simulink model "control_foc"  (R2023b)
settings: Solver=FixedStepDiscrete  StartTime=0.0  StopTime=10.0  FixedStep=ControlFOC_Ts  RelTol=1e-3  EnableMultiTasking=on
model workspace (MAT data in the model file):
  ControlFOC_Ts = Simulink.Parameter
  ControlFOC_Ts.Value = 3.65714285714e-05
  ControlFOC_Ts.DataType = 'auto'
  ControlFOC_Ts.DocUnits = 's'
  ControlFOC_Ts.Complexity = 'real'
  ControlFOC_Ts.Dimensions = [1 1]
libraries: mcbcontrolslib x4, slpidlib x2, dspstat3 x2, simulink x1
settings Model: DataDictionary=EmbeddedBoardDD.sldd  Creator=ascalzo  LastModifiedBy=mfussi
settings SolverCC: AllowMultiTaskInputOutput=on  AutoInsertRateTranBlk=on  InsertRTBMode=Never (minimum delay)
settings DataIOCC: SaveOutput=off  SignalLogging=off  DSMLogging=off  SaveTime=off  ReturnWorkspaceOutputs=off
settings OptimizationCC: DefaultParameterBehavior=Inlined  DefaultUnderspecifiedDataType=single  StrengthReduction=on  PassReuseOutputArgsAs=Individual arguments  OptimizeBlockOrder=speed  OptimizationPriority=Speed  OptimizationCustomize=off  MultiThreadedLoops=on  EfficientTunableParamExpr=on
settings DebuggingCC: ParameterPrecisionLossMsg=none  UnconnectedInputMsg=warning  UnconnectedOutputMsg=warning  UnconnectedLineMsg=warning
settings HardwareCC: ProdBitPerPointer=32  ProdBitPerSizeT=32  ProdBitPerPtrDiffT=32  ProdLargestAtomicInteger=Long  ProdLargestAtomicFloat=Double  ProdWordSize=32  ProdHWDeviceType=ARM Compatible->ARM Cortex-M
settings ModelReferenceCC: UpdateModelReferenceTargets=Force  EnableRefExpFcnMdlSchedulingChecks=on
settings SFSimCC: MATLABDynamicMemAlloc=off
settings RTWCC: Description=Embedded Coder  SystemTargetFile=ert.tlc  GenCodeOnly=on  PackageGeneratedCodeAndArtifacts=on  PackageName=control_foc  TemplateMakefile=ert_default_tmf  TargetLang=C++  DLArmComputeVersion=19.05
settings CodeAppCC: ForceParamTrailComments=on  IgnoreCustomStorageClasses=off  MaxIdLength=60  OperatorAnnotations=on  SimulinkDataObjDesc=on  SFDataObjDesc=on  InsertBlockDesc=on
settings ERTTargetCC: TargetLangStandard=C++03 (ISO)  CodeReplacementLibrary=ARM Cortex-M,iCubTech  GenerateSampleERTMain=on  CodeInterfacePackaging=Reusable function  InlinedParameterPlacement=NonHierarchical  RootIOFormat=Structure reference  ERTCustomFileTemplate=example_file_process.tlc

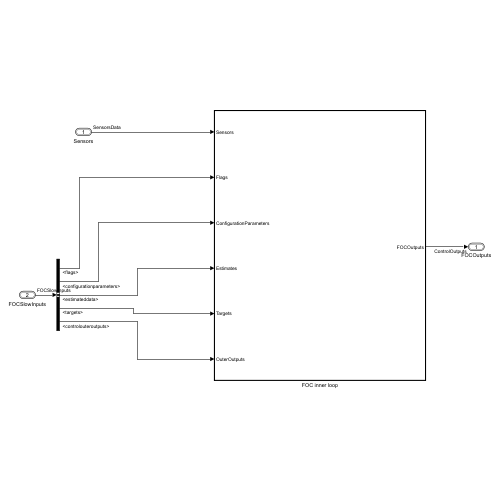
[thumbnail: Simulink's stored preview of the top-level diagram]
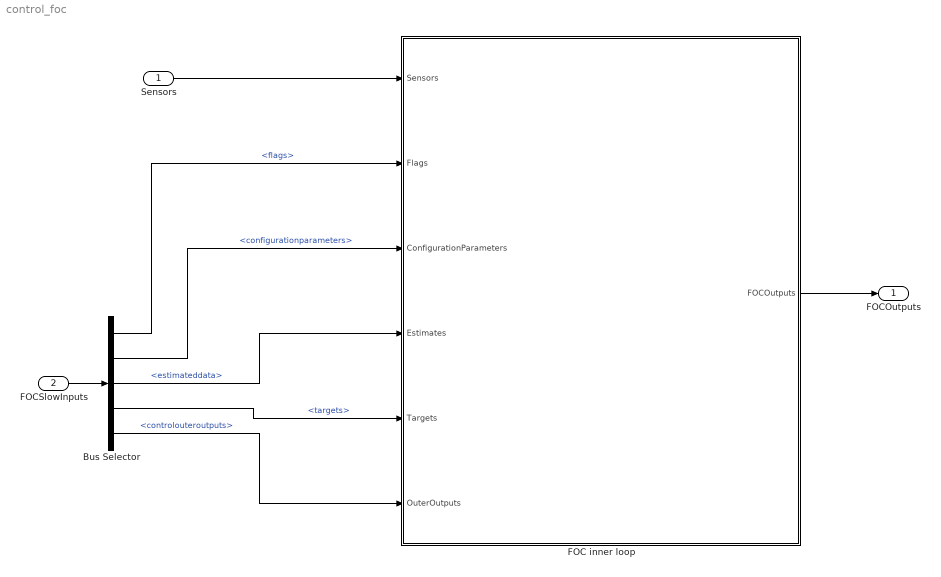
== system control_foc ==
  Sensors : Inport  OutDataTypeStr=Bus: SensorsData  BusOutputAsStruct=on
  FOCSlowInputs : Inport  Port=2  OutDataTypeStr=Bus: FOCSlowInputs  BusOutputAsStruct=on
  Bus Selector : BusSelector  OutputSignals=flags,configurationparameters,estimateddata,targets,controlouteroutputs
  FOC inner loop : Subsystem  TreatAsAtomicUnit=on  RTWFcnName=FOCInnerLoop
      settings: RTWFcnNameOpts=User specified  RTWFileNameOpts=Use function name  FunctionInterfaceSpec=Allow arguments (Optimized)
  FOCOutputs : Outport  OutDataTypeStr=Bus: ControlOutputs  BusOutputAsStruct=on
  wires:
  FOC inner loop/1(FOCOutputs) -> FOCOutputs/1
  FOCSlowInputs/1 -> Bus Selector/1
  Bus Selector/1 -> FOC inner loop/2(Flags)  "<flags>"
  Bus Selector/2 -> FOC inner loop/3(ConfigurationParameters)  "<configurationparameters>"
  Bus Selector/3 -> FOC inner loop/4(Estimates)  "<estimateddata>"
  Bus Selector/4 -> FOC inner loop/5(Targets)  "<targets>"
  Bus Selector/5 -> FOC inner loop/6(OuterOutputs)  "<controlouteroutputs>"
  Sensors/1 -> FOC inner loop/1(Sensors)

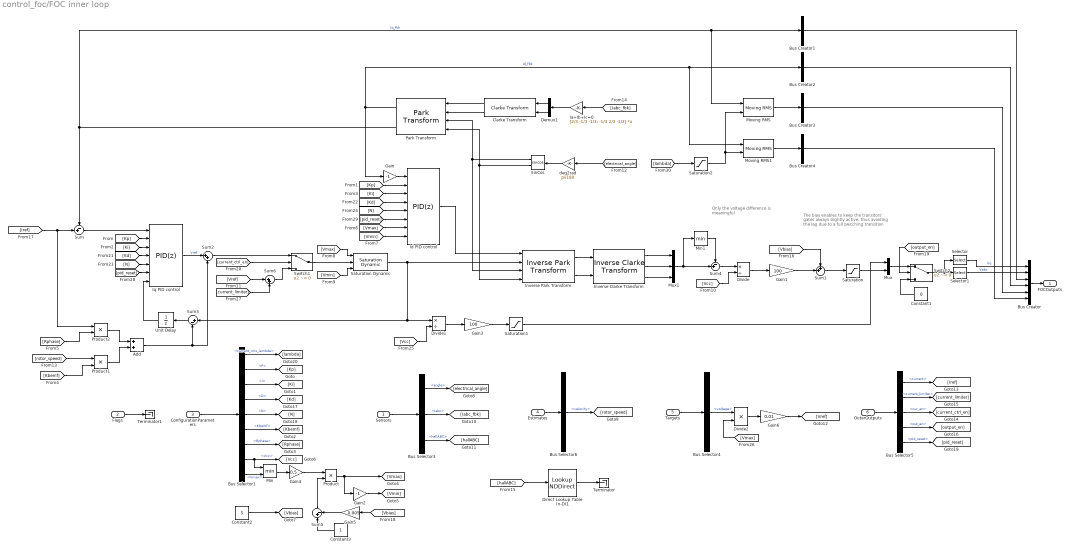
== system control_foc/FOC inner loop ==
  note: Only the voltage difference
      | is meaningful
  note: The bias enables to keep the transitors'
      | gates always slightly active, thus avoiding
      | the lag due to a full switching transition
  Sensors : Inport  OutDataTypeStr=Bus: SensorsData
  Flags : Inport  Port=2  OutDataTypeStr=Bus: Flags
  ConfigurationParameters : Inport  Port=3  OutDataTypeStr=Bus: ConfigurationParameters
  Estimates : Inport  Port=4  OutDataTypeStr=Bus: EstimatedData
  Targets : Inport  Port=5  OutDataTypeStr=Bus: Targets
  OuterOutputs : Inport  Port=6  OutDataTypeStr=Bus: ControlOuterOutputs
  Add : Sum
  Bus Creator : BusCreator  Inputs=6  OutDataTypeStr=Bus: ControlOutputs  NonVirtualBus=on
      settings: InheritFromInputs=off
  Bus Creator{1..4} (4 alike) : BusCreator  Inputs=1  OutDataTypeStr=Bus: MotorCurrent  NonVirtualBus=on
      settings: InheritFromInputs=off
  Bus Selector1 : BusSelector  OutputSignals=estimationconfig.current_rms_lambda,CurLoopPID.P,CurLoopPID.I,CurLoopPID.D,CurLoopPID.N,motorconfig.Kbemf,motorconfig.Rphase,motorconfig.Vcc,motorconfig.Vmax
  Bus Selector3 : BusSelector  OutputSignals=motorsensors.angle,motorsensors.Iabc,motorsensors.hallABC
  Bus Selector4 : BusSelector  OutputSignals=motorvoltage.voltage
  Bus Selector5 : BusSelector  OutputSignals=motorcurrent.current,current_limiter,cur_en,out_en,pid_reset
  Bus Selector6 : BusSelector  OutputSignals=jointvelocities.velocity
  Clarke Transform : mcbcontrolslib/Clarke Transform  VariantControl=Variant2  PhaseInput=Two inputs  EnPowerInv=off
  Constant1 : Constant  Value=0  OutDataTypeStr=single
  Constant2 : Constant  Value=5  OutDataTypeStr=single
  Constant3 : Constant  OutDataTypeStr=single
  Demux1 : Demux  Outputs=2
  Direct Lookup Table (n-D)1 : LookupNDDirect  NumberOfTableDimensions=1  Table=[-1,270,150,210,30,330,90,-1]  RemoveProtectionInput=on  TableDataTypeStr=single
  Divide : Product  Inputs=*/
  Divide1 : Product  Inputs=*/
  Divide2 : Product
  Gain : Gain  Gain=-1
  Gain1 : Gain  Gain=100
  Gain2 : Gain  Gain=-1
  Gain3 : Gain  Gain=100
  Gain4 : Gain  Gain=0.5
  Gain5 : Gain  Gain=0.005
  Gain6 : Gain  Gain=0.01
  Ia+Ib+Ic=0 : Gain  Gain=[2/3 -1/3 -1/3; -1/3 2/3 -1/3]  Multiplication=Matrix(K*u) (u vector)
  Id PID control : slpidlib/PID Controller  Controller=PID  Form=Parallel  TimeDomain=Discrete-time  UseExternalTs=off  SampleTime=-1  IntegratorMethod=Trapezoidal  FilterMethod=Trapezoidal  ControllerParametersSource=external  P=1  I=1  UseKiTs=off  D=0  N=100  UseFilter=on  TunerSelectOption=Frequency Response Based  InitialConditionSource=internal  InitialConditionForIntegrator=0  InitialConditionForFilter=0  DifferentiatorICPrevScaledInput=0  ExternalReset=rising  TrackingMode=off  Kt=1  LimitOutput=on  SatLimitsSource=external  UpperSaturationLimit=100  LowerSaturationLimit=-100  LinearizeAsGain=on  AntiWindupMode=clamping  Kb=1  LimitIntegrator=off  UpperIntegratorSaturationLimit=inf  LowerIntegratorSaturationLimit=-inf  POutMin=[]  POutMax=[]  IOutMin=[]  IOutMax=[]  DOutMin=[]  DOutMax=[]  NOutMin=[]  NOutMax=[]  SumOutMin=[]  SumOutMax=[]  SaturationOutMin=[]  SaturationOutMax=[]  PParamMin=[]  PParamMax=[]  IParamMin=[]  IParamMax=[]  DParamMin=[]  DParamMax=[]  NParamMin=[]  NParamMax=[]  KbParamMin=[]  KbParamMax=[]  KtParamMin=[]  KtParamMax=[]  KbOutMin=[]  KbOutMax=[]  KtOutMin=[]  KtOutMax=[]  IntegratorOutMin=[]  IntegratorOutMax=[]  FilterOutMin=[]  FilterOutMax=[]  SumI1OutMin=[]  SumI1OutMax=[]  SumI2OutMin=[]  SumI2OutMax=[]  SumI3OutMin=[]  SumI3OutMax=[]  SumI4OutMin=[]  SumI4OutMax=[]  SumDOutMin=[]  SumDOutMax=[]  DifferentiatorOutMin=[]  DifferentiatorOutMax=[]  FilterDiffOutCoefMin=[]  FilterDiffOutCoefMax=[]  ReciprocalOutMin=[]  ReciprocalOutMax=[]  SumDenOutMin=[]  SumDenOutMax=[]  SumNumOutMin=[]  SumNumOutMax=[]  DivideOutMin=[]  DivideOutMax=[]  UdiffTsProdOutMin=[]  UdiffTsProdOutMax=[]  NTsProdOutMin=[]  NTsProdOutMax=[]  UintegralTsProdOutMin=[]  UintegralTsProdOutMax=[]  UngainTsProdOutMin=[]  UngainTsProdOutMax=[]  ClampingZeroOutDataTypeStr=Inherit: Inherit via back propagation  ClampingZeroOutMin=[]  ClampingZeroOutMax=[]  FilterDenConstantOutDataTypeStr=Inherit: Inherit via back propagation  FilterDenConstantOutMin=[]  FilterDenConstantOutMax=[]  PCopyOutDataTypeStr=Inherit: Inherit via back propagation  PCopyOutMin=[]  PCopyOutMax=[]  NCopyOutDataTypeStr=Inherit: Inherit via back propagation  NCopyOutMin=[]  NCopyOutMax=[]  IntegratorContinuousStateAttributes=''  IntegratorStateMustResolveToSignalObject=off  IntegratorRTWStateStorageClass=Auto  FilterContinuousStateAttributes=''  FilterStateMustResolveToSignalObject=off  FilterRTWStateStorageClass=Auto  ParallelPVariant=ExternalParameters  IdealPVariant=Disabled  IVariant=ExternalParameters  DVariant=ExternalParameters  IntegratorVariant=Discrete  SatVariant=External  AWVariant=DiscClampingParallel  PCopyVariant=Disabled  TRVariant=Disabled  FdbkBlocksVariant=Feedback  IdealPFdbkVariant=Passthrough  SatFdbkVariant=Passthrough  DerivativeFilterVariant=TrapezoidalFilter  NVariant=ExternalParameters  NCopyVariant=ExternalParameters  FilterICVariant=InternalICsFilter  IntegratorICVariant=InternalICs  ExternalResetVariant=ExternalReset  TRSumVariant=Passthrough  SumFdbkVariant=Enabled  SumVariant=Sum_PID  TsampFilterVariant=InternalTs  TsampNgainVariant=Passthrough  TsampIntegralVariant=Disabled_SignalSpec  ExternalSaturationOutDataTypeStr=Inherit: Same as second input
  Inverse Clarke Transform : mcbcontrolslib/Inverse Clarke Transform  PhaseInput=Two inputs  EnPowerInv=off
  Inverse Park Transform : mcbcontrolslib/Inverse Park Transform  PhaseInput=Two inputs  AxisAlignment=Q-axis  ThetaInput=Sine and Cosine electrical position  AngleInput=Per-unit  N_points=1024
  Iq PID control : slpidlib/PID Controller  Controller=PID  Form=Parallel  TimeDomain=Discrete-time  UseExternalTs=off  SampleTime=-1  IntegratorMethod=Trapezoidal  FilterMethod=Trapezoidal  ControllerParametersSource=external  P=1  I=1  UseKiTs=off  D=0  N=100  UseFilter=on  TunerSelectOption=Frequency Response Based  InitialConditionSource=internal  InitialConditionForIntegrator=0  InitialConditionForFilter=0  DifferentiatorICPrevScaledInput=0  ExternalReset=rising  TrackingMode=on  Kt=1  LimitOutput=off  SatLimitsSource=internal  UpperSaturationLimit=100  LowerSaturationLimit=-100  LinearizeAsGain=on  AntiWindupMode=clamping  Kb=1  LimitIntegrator=off  UpperIntegratorSaturationLimit=inf  LowerIntegratorSaturationLimit=-inf  POutMin=[]  POutMax=[]  IOutMin=[]  IOutMax=[]  DOutMin=[]  DOutMax=[]  NOutMin=[]  NOutMax=[]  SumOutMin=[]  SumOutMax=[]  SaturationOutMin=[]  SaturationOutMax=[]  PParamMin=[]  PParamMax=[]  IParamMin=[]  IParamMax=[]  DParamMin=[]  DParamMax=[]  NParamMin=[]  NParamMax=[]  KbParamMin=[]  KbParamMax=[]  KtParamMin=[]  KtParamMax=[]  KbOutMin=[]  KbOutMax=[]  KtOutMin=[]  KtOutMax=[]  IntegratorOutMin=[]  IntegratorOutMax=[]  FilterOutMin=[]  FilterOutMax=[]  SumI1OutMin=[]  SumI1OutMax=[]  SumI2OutMin=[]  SumI2OutMax=[]  SumI3OutMin=[]  SumI3OutMax=[]  SumI4OutMin=[]  SumI4OutMax=[]  SumDOutMin=[]  SumDOutMax=[]  DifferentiatorOutMin=[]  DifferentiatorOutMax=[]  FilterDiffOutCoefMin=[]  FilterDiffOutCoefMax=[]  ReciprocalOutMin=[]  ReciprocalOutMax=[]  SumDenOutMin=[]  SumDenOutMax=[]  SumNumOutMin=[]  SumNumOutMax=[]  DivideOutMin=[]  DivideOutMax=[]  UdiffTsProdOutMin=[]  UdiffTsProdOutMax=[]  NTsProdOutMin=[]  NTsProdOutMax=[]  UintegralTsProdOutMin=[]  UintegralTsProdOutMax=[]  UngainTsProdOutMin=[]  UngainTsProdOutMax=[]  ClampingZeroOutDataTypeStr=Inherit: Inherit via back propagation  ClampingZeroOutMin=[]  ClampingZeroOutMax=[]  FilterDenConstantOutDataTypeStr=Inherit: Inherit via back propagation  FilterDenConstantOutMin=[]  FilterDenConstantOutMax=[]  PCopyOutDataTypeStr=Inherit: Inherit via back propagation  PCopyOutMin=[]  PCopyOutMax=[]  NCopyOutDataTypeStr=Inherit: Inherit via back propagation  NCopyOutMin=[]  NCopyOutMax=[]  IntegratorContinuousStateAttributes=''  IntegratorStateMustResolveToSignalObject=off  IntegratorRTWStateStorageClass=Auto  FilterContinuousStateAttributes=''  FilterStateMustResolveToSignalObject=off  FilterRTWStateStorageClass=Auto  ParallelPVariant=ExternalParameters  IdealPVariant=Disabled  IVariant=ExternalParameters  DVariant=ExternalParameters  IntegratorVariant=Discrete  SatVariant=Disabled  AWVariant=Passthrough  PCopyVariant=Disabled  TRVariant=Enabled  FdbkBlocksVariant=Feedback  IdealPFdbkVariant=Passthrough  SatFdbkVariant=Passthrough  DerivativeFilterVariant=TrapezoidalFilter  NVariant=ExternalParameters  NCopyVariant=ExternalParameters  FilterICVariant=InternalICsFilter  IntegratorICVariant=InternalICs  ExternalResetVariant=ExternalReset  TRSumVariant=TrackingMode  SumFdbkVariant=Enabled  SumVariant=Sum_PID  TsampFilterVariant=InternalTs  TsampNgainVariant=Passthrough  TsampIntegralVariant=Disabled_SignalSpec  ExternalSaturationOutDataTypeStr=Inherit: Same as second input
  Min : MinMax  Inputs=2
  Min1 : MinMax
  Moving RMS : dspstat3/Moving RMS  Method=Exponential weighting  ForgettingFactorPort=on  SpecifyWindowLength=on  WindowLength=4  OverlapLength=3  AllowArbitraryInputLength=off  ForgettingFactor=1  SimulateUsing=Code generation
  Moving RMS1 : dspstat3/Moving RMS  Method=Exponential weighting  ForgettingFactorPort=on  SpecifyWindowLength=on  WindowLength=4  OverlapLength=3  AllowArbitraryInputLength=off  ForgettingFactor=1  SimulateUsing=Code generation
  Mux : Mux  Inputs=2
  Mux1 : Mux  Inputs=3
  Park Transform : mcbcontrolslib/Park Transform  PhaseInput=Two inputs  AxisAlignment=Q-axis  ThetaInput=Sine and Cosine electrical position  AngleInput=Per-unit  N_points=1024
  Product : Product
  Product1 : Product
  Product2 : Product
  Saturation : Saturate  UpperLimit=100  LowerLimit=0
  Saturation Dynamic : simulink/Discontinuities/Saturation Dynamic  OutMin=[]  OutMax=[]  OutDataTypeStr=Inherit: Same as second input  OutDataType=fixdt(1, 16)  OutScaling=2^-10  DoSatur=off
  Saturation1 : Saturate  UpperLimit=100  LowerLimit=-100
  Saturation2 : Saturate  UpperLimit=1  LowerLimit=0
  Selector : Selector  InputPortWidth=4  IndexOptions=Index vector (dialog)  Indices=1  OutputSizes=1
  Selector1 : Selector  InputPortWidth=4  IndexOptions=Index vector (dialog)  Indices=[2 3 4]  OutputSizes=1
  SinCos : Trigonometry  Operator=sincos
  Sum : Sum  Inputs=-+|
  Sum1 : Sum  Inputs=++|
  Sum2 : Sum  Inputs=|++
  Sum3 : Sum  Inputs=|+-
  Sum4 : Sum  Inputs=-+|
  Sum5 : Sum  Inputs=|+-
  Sum6 : Sum  Inputs=|++
  Switch1 : Switch  Criteria=u2 ~= 0  SaturateOnIntegerOverflow=off  InputSameDT=off
  Switch2 : Switch  Criteria=u2 ~= 0  SaturateOnIntegerOverflow=off  InputSameDT=off
  Terminator : Terminator
  Terminator1 : Terminator
  Unit Delay : UnitDelay  SampleTime=-1  HasFrameUpgradeWarning=on
  deg2rad : Gain  Gain=pi/180
  FOCOutputs : Outport  OutDataTypeStr=Bus: ControlOutputs
  wires:
  Sum/1 -> Iq PID control/1
  [current_ctrl_en] -> Switch1/2
  Park Transform/1 -> Gain/1, Moving RMS1/1, Bus Creator2/1  "Id_fbk"
  Gain/1 -> Id PID control/1
  Park Transform/2 -> Sum/1, Moving RMS/1, Bus Creator1/1  "Iq_fbk"
  [Kp] -> Iq PID control/2
  [Ki] -> Iq PID control/3
  [Kp] -> Id PID control/2
  [Ki] -> Id PID control/3
  Constant1/1 -> Switch2/3
  Clarke Transform/1 -> Park Transform/1
  Clarke Transform/2 -> Park Transform/2
  SinCos/1 -> Inverse Park Transform/3, Park Transform/3
  Inverse Clarke Transform/1 -> Mux1/1
  Inverse Clarke Transform/2 -> Mux1/2
  Inverse Clarke Transform/3 -> Mux1/3
  Inverse Park Transform/1 -> Inverse Clarke Transform/1
  Inverse Park Transform/2 -> Inverse Clarke Transform/2
  Id PID control/1 -> Inverse Park Transform/1
  SinCos/2 -> Inverse Park Transform/4, Park Transform/4
  Add/1 -> Sum3/2, Sum2/2
  [Iref] -> Product2/1, Sum/2
  Product2/1 -> Add/1
  Iq PID control/1 -> Sum2/1  "Vref"
  Sum3/1 -> Unit Delay/1
  Product1/1 -> Add/2
  [rotor_speed] -> Product1/1
  [Kbemf] -> Product1/2
  Bus Selector1/7 -> [Rphase]  "<Rphase>"
  [Rphase] -> Product2/2
  Unit Delay/1 -> Iq PID control/7
  [Vmax] -> Id PID control/7
  [Vmin] -> Id PID control/8
  [Vmax] -> Saturation Dynamic/1
  [Vmin] -> Saturation Dynamic/3
  Bus Selector1/8 -> [Vcc], Min/1  "<Vcc>"
  Divide/1 -> Gain1/1
  [Vcc] -> Divide/2
  [Iabc_fbk] -> Ia+Ib+Ic=0/1
  Ia+Ib+Ic=0/1 -> Demux1/1
  Demux1/1 -> Clarke Transform/1
  Demux1/2 -> Clarke Transform/2
  deg2rad/1 -> SinCos/1
  [electrical_angle] -> deg2rad/1
  Bus Creator/1 -> FOCOutputs/1
  ConfigurationParameters/1 -> Bus Selector1/1
  Sensors/1 -> Bus Selector3/1
  Bus Selector3/1 -> [electrical_angle]  "<angle>"
  Bus Selector3/2 -> [Iabc_fbk]  "<Iabc>"
  Targets/1 -> Bus Selector4/1
  OuterOutputs/1 -> Bus Selector5/1
  Bus Selector5/1 -> [Iref]  "<current>"
  Bus Selector5/3 -> [current_ctrl_en]  "<cur_en>"
  Bus Selector5/4 -> [output_en]  "<out_en>"
  [output_en] -> Switch2/2
  Estimates/1 -> Bus Selector6/1
  Bus Selector6/1 -> [rotor_speed]  "<velocity>"
  Bus Selector3/3 -> [hallABC]  "<hallABC>"
  [hallABC] -> Direct Lookup Table (n-D)1/1
  Direct Lookup Table (n-D)1/1 -> Terminator/1
  [Kd] -> Iq PID control/4
  [Kd] -> Id PID control/4
  [N] -> Iq PID control/5
  [N] -> Id PID control/5
  Bus Creator1/1 -> Bus Creator/3
  Sum2/1 -> Switch1/1
  Switch1/1 -> Saturation Dynamic/2
  Saturation Dynamic/1 -> Sum3/1, Divide1/1, Inverse Park Transform/2
  [Vcc] -> Divide1/2
  Divide1/1 -> Gain3/1
  Gain3/1 -> Saturation1/1
  Sum1/1 -> Saturation/1
  Gain1/1 -> Sum1/2
  [Vbias] -> Sum1/1
  Min/1 -> Gain4/1
  Bus Selector1/9 -> Min/2  "<Vmax>"
  Gain4/1 -> Product/1
  Sum4/1 -> Divide/1
  Mux1/1 -> Min1/1, Sum4/2
  Min1/1 -> Sum4/1
  Constant2/1 -> [Vbias]
  [Vbias] -> Gain5/1
  Product/1 -> Gain2/1, [Vmax]
  Gain2/1 -> [Vmin]
  Sum5/1 -> Product/2
  Constant3/1 -> Sum5/1
  Gain5/1 -> Sum5/2
  Bus Selector4/1 -> Divide2/1  "<voltage>"
  Divide2/1 -> Gain6/1
  [Vmax] -> Divide2/2
  Gain6/1 -> [Vref]
  Bus Selector5/2 -> [current_limiter]  "<current_limiter>"
  Sum6/1 -> Switch1/3
  [Vref] -> Sum6/1
  [current_limiter] -> Sum6/2
  Bus Selector1/2 -> [Kp]  "<P>"
  Bus Selector1/3 -> [Ki]  "<I>"
  Bus Selector1/4 -> [Kd]  "<D>"
  Bus Selector1/5 -> [N]  "<N>"
  Bus Selector1/6 -> [Kbemf]  "<Kbemf>"
  Saturation/1 -> Mux/2
  Saturation1/1 -> Mux/1
  Mux/1 -> Switch2/1
  Switch2/1 -> Selector/1, Selector1/1
  Selector/1 -> Bus Creator/1  "Vq"
  Selector1/1 -> Bus Creator/2  "Vabc"
  Bus Selector5/5 -> [pid_reset]  "<pid_reset>"
  [pid_reset] -> Iq PID control/6
  [pid_reset] -> Id PID control/6
  Flags/1 -> Terminator1/1
  Bus Creator2/1 -> Bus Creator/4
  Moving RMS/1 -> Bus Creator3/1
  Moving RMS1/1 -> Bus Creator4/1
  Bus Creator3/1 -> Bus Creator/5
  Bus Creator4/1 -> Bus Creator/6
  Saturation2/1 -> Moving RMS/2, Moving RMS1/2
  Bus Selector1/1 -> [lambda]  "<current_rms_lambda>"
  [lambda] -> Saturation2/1
